simulink model "Windkessel"  (R2023b)
settings: Solver=VariableStepAuto  StartTime=0.0  StopTime=4  MaxStep=t_end_cyc/resolution  RelTol=1e-3
values from neighbouring files (symbols this model uses):
  C = [1,NaN,NaN;1,1.75,5.16;1,1.22,2.53]    [i_Windkessel_Input_Current.m]
  L = [NaN,NaN,NaN;NaN,NaN,NaN;0.005,0.0051,0.0054]    [i_Windkessel_Input_Current.m]
  R = [1,NaN,NaN;1,0.79,0.63;1,0.79,0.63]    [i_Windkessel_Input_Current.m]
  r = [NaN,NaN,NaN;0.05,0.033,0.03;0.05,0.056,0.045]    [i_Windkessel_Input_Current.m]
libraries: simulink x1
settings Model: Creator=n8dsa  LastModifiedBy=n8dsa

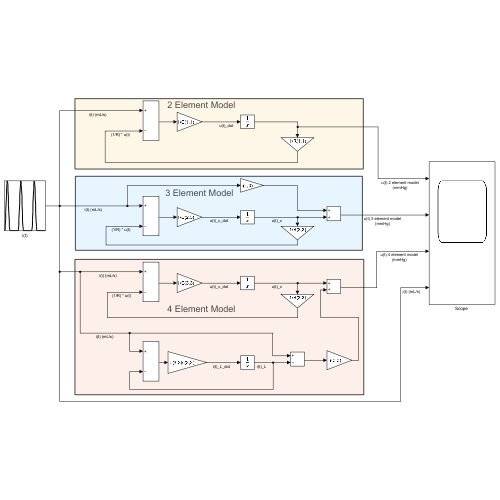
[thumbnail: Simulink's stored preview of the top-level diagram]
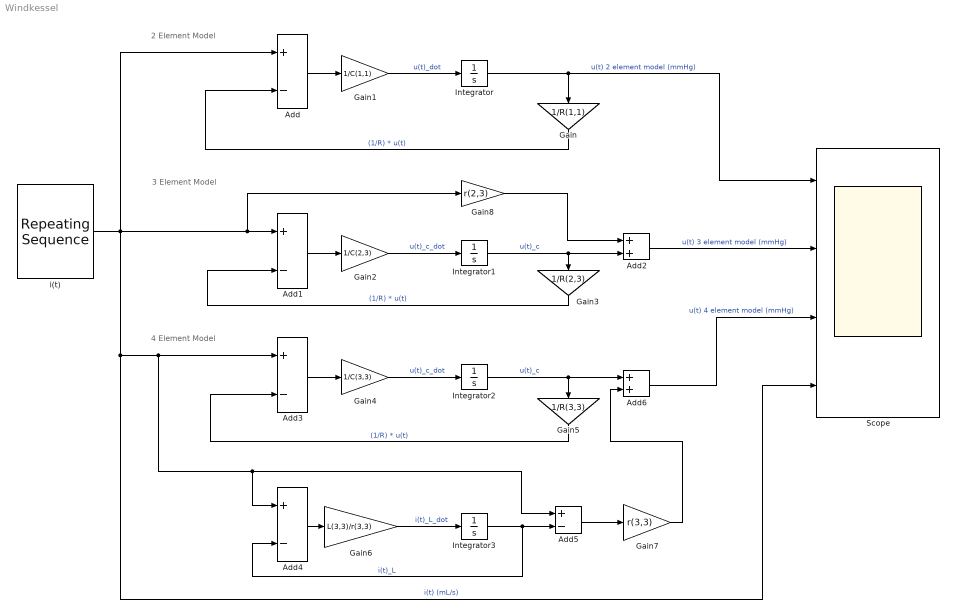
== system Windkessel ==
  note: 4 Element Model
  note: 3 Element Model
  note: 2 Element Model
  Add{,1,3..5} (5 alike) : Sum  Inputs=+-
  Add2 : Sum
  Add6 : Sum
  Gain : Gain  Gain=1/R(1,1)
  Gain1 : Gain  Gain=1/C(1,1)
  Gain2 : Gain  Gain=1/C(2,3)
  Gain3 : Gain  Gain=1/R(2,3)
  Gain4 : Gain  Gain=1/C(3,3)
  Gain5 : Gain  Gain=1/R(3,3)
  Gain6 : Gain  Gain=L(3,3)/r(3,3)
  Gain7 : Gain  Gain=r(3,3)
  Gain8 : Gain  Gain=r(2,3)
  Integrator{,1..3} (4 alike) : Integrator
  "Scope " : Scope  NumInputPorts=4
  i(t) : simulink/Sources/Repeating Sequence  rep_seq_t=t  rep_seq_y=i
  wires:
  i(t)/1 -> Add5/1, Add4/1, Add3/1, "Scope "/4, Gain8/1, Add1/1, Add/1  "i(t) (mL/s)"
  Gain1/1 -> Integrator/1  "u(t)_dot"
  Integrator/1 -> Gain/1, "Scope "/1  "u(t) 2 element model (mmHg)"
  Gain/1 -> Add/2  "(1/R) * u(t)"
  Add/1 -> Gain1/1
  Gain2/1 -> Integrator1/1  "u(t)_c_dot"
  Integrator1/1 -> Add2/2, Gain3/1  "u(t)_c"
  Add1/1 -> Gain2/1
  Gain3/1 -> Add1/2  "(1/R) * u(t)"
  Add2/1 -> "Scope "/2  "u(t) 3 element model (mmHg)"
  Gain4/1 -> Integrator2/1  "u(t)_c_dot"
  Integrator2/1 -> Add6/1, Gain5/1  "u(t)_c"
  Add3/1 -> Gain4/1
  Gain5/1 -> Add3/2  "(1/R) * u(t)"
  Gain6/1 -> Integrator3/1  "i(t)_L_dot"
  Integrator3/1 -> Add5/2, Add4/2  "i(t)_L"
  Add4/1 -> Gain6/1
  Add5/1 -> Gain7/1
  Gain7/1 -> Add6/2
  Add6/1 -> "Scope "/3  "u(t) 4 element model (mmHg)"
  Gain8/1 -> Add2/1
